simulink model "c166_ccp"  (Simulink 6.0)
settings: Solver=FixedStepDiscrete  StartTime=0.0  StopTime=16  FixedStep=0.01  RelTol=1e-3
PreLoadFcn:
  | c166_ccp_data
values from neighbouring files (symbols this model uses):
  STEP_PARAM = Simulink.Parameter    [c166_ccp_data.m]
undefined symbols (not defined in the file or in its folder): c166rt_ccp, Target_CCP
libraries: c166drivers x2
CloseFcn:
  | rtwprivate ssgencode ModelCloseRequest c166rt_ccp
settings Model: Creator=The MathWorks Inc.  LastModifiedBy=batserve  ExtModeAutoUpdateStatusClock=off  ProdHWDeviceType=Infineon C16x
settings DataIOCC: SignalLoggingName=logsOut
settings OptimizationCC: InlineParams=on  ZeroExternalMemoryAtStartup=off  ZeroInternalMemoryAtStartup=off  InitFltsAndDblsToZero=off  LifeSpan=1
settings DebuggingCC: CheckExecutionContextPreStartOutputMsg=on  CheckExecutionContextRuntimeOutputMsg=on  SignalResolutionControl=UseLocalSettings  SolverPrmCheckMsg=none
settings HardwareCC: ProdBitPerInt=16  ProdEndianess=LittleEndian  ProdWordSize=16  ProdHWDeviceType=Infineon C16x  TargetHWDeviceType=32-bit Generic
settings ModelReferenceCC: UpdateModelReferenceTargets=IfOutOfDate
settings RTWCC: SystemTargetFile=c166.tlc  TemplateMakefile=c166.tmf  ProcessScript=c166_make_rtw_hook
settings CodeAppCC: IgnoreCustomStorageClasses=off
settings STFCustomTargetCC: TargetFcnLib=ansi_tfl_tmw.mat  GenFloatMathFcnCalls=ANSI_C  GenerateSampleERTMain=on  CombineOutputUpdateFcns=on  ERTCustomFileBanners=on  SupportNonFinite=off  SystemTargetFile=c166.tlc
settings ERTTargetCC: TargetFcnLib=ansi_tfl_tmw.mat  GenFloatMathFcnCalls=ANSI_C  GenerateSampleERTMain=on  SupportNonFinite=off  SupportContinuousTime=on  SupportNonInlinedSFcns=on  GenerateASAP2=on  RootIOFormat=Individual Arguments  ERTCustomFileTemplate=example_file_process.tlc  InitialValueSource=Model
settings CustomProperty: DataType=RTWOptions_EnumType__toolbox_rtw_targets_c166_c166_c166_BuildActionC166  Value=None
settings EnumStrPairs: String=Run_with_simulator

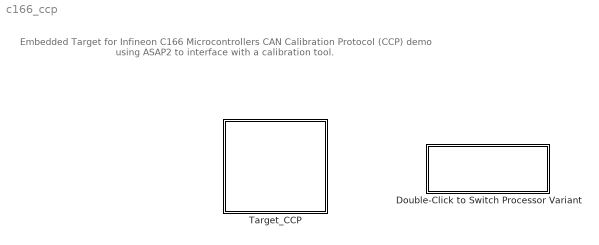
== system c166_ccp ==
  note: Embedded Target for Infineon C166 Microcontrollers
      | CAN Calibration Protocol (CCP) demo using
      | ASAP2 to interface with a calibration tool.
  Double-Click to Switch Processor Variant : Subsystem  PropExecContextAcrossSSBoundary=on
      settings: OpenFcn=c166switchconfig(gcs)
      mask Display: disp('Switch Target\nProcessor Variant');
  Target_CCP : Subsystem  InitFcn=|  PropExecContextAcrossSSBoundary=on
      | % START RTW CONFIGURATION CODE %
      | RTWConfigurationCB('rtw_target_initfcn',gcb);
      | % END RTW CONFIGURATION CODE %
      mask Display: image(imread('target_affordance_icon.jpg'),'bottom-right')

== system c166_ccp/Double-Click to Switch Processor Variant ==

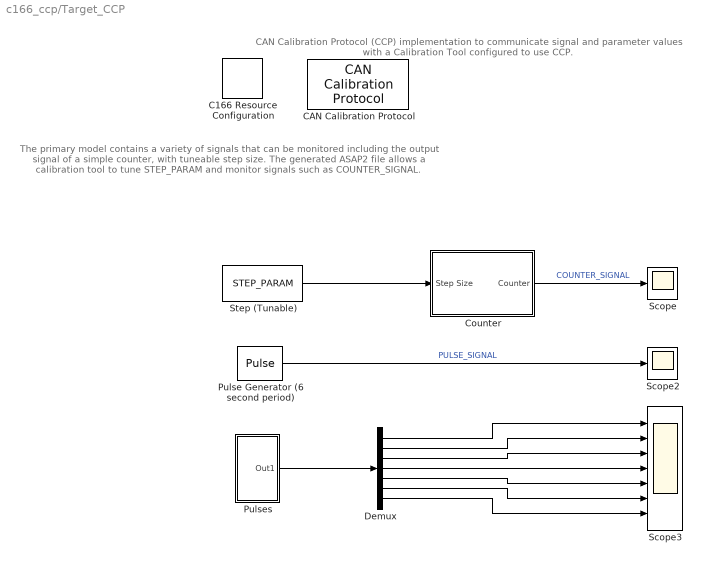
== system c166_ccp/Target_CCP ==
  note: The primary model contains a variety of signals that can be monitored
      | including the output signal of a simple counter, with tuneable
      | step size. The generated ASAP2 file allows a calibration tool to tune
      | STEP_PARAM and monitor signals such as COUNTER_SIGNAL.
  note: CAN Calibration Protocol (CCP) implementation
      | to communicate signal and parameter values
      |  with a Calibration Tool configured to use CCP.
  C166 Resource Configuration : c166drivers/C166 Resource Configuration  Tag=RTW CONFIGURATION BLOCK  Priority=-100000  oldParentName=c166rt_ccp/Target_CCP  oldBlockName=|  defaultConfigLibrary=c166drivers
      | c166rt_ccp/Target_CCP/C166
      | Resource
      | Configuration
  CAN Calibration Protocol : c166drivers/CAN Interface/CAN Calibration Protocol  CCP_STATION_ID=hex2dec('1')  module=A  ccp_cro_id=hex2dec('6FA')  ccp_cro_message_type=Extended (29-bit identifier)  ccp_return_id=hex2dec('6FB')  ccp_return_message_type=Extended (29-bit identifier)  TOTAL_NUM_ODTS=8  cro_sample_time=0.01
  Counter : Subsystem  PropExecContextAcrossSSBoundary=on
  Demux : Demux  Outputs=7
  Pulse Generator (6 second period) : DiscretePulseGenerator  Amplitude=uint16(60000)  Period=12  PulseWidth=4  SampleTime=0.5
  Pulses : Subsystem  PropExecContextAcrossSSBoundary=on
  Scope : Scope
      settings: YMin=-130  YMax=0
  Scope2 : Scope
      settings: YMin=-130  YMax=0  SaveName=ScopeData2
  Scope3 : Scope  NumInputPorts=7
      settings: YMin=-130~-5~-5~-5~-5~-5~-5  YMax=0~5~5~5~5~5~5  SaveName=ScopeData3
  Step (Tunable) : Constant  Value=STEP_PARAM
  wires:
  Step (Tunable)/1 -> Counter/1(Step Size)
  Counter/1(Counter) -> Scope/1  "COUNTER_SIGNAL"
  Pulse Generator (6 second period)/1 -> Scope2/1  "PULSE_SIGNAL"
  Pulses/1(Out1) -> Demux/1
  Demux/1 -> Scope3/1
  Demux/2 -> Scope3/2
  Demux/3 -> Scope3/3
  Demux/4 -> Scope3/4
  Demux/5 -> Scope3/5
  Demux/6 -> Scope3/6
  Demux/7 -> Scope3/7

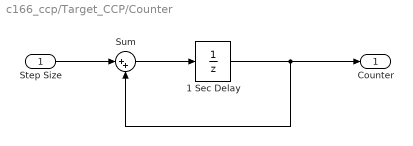
== system c166_ccp/Target_CCP/Counter ==
  Step Size : Inport  Port=1  LatchInput=off
  1 Sec Delay : UnitDelay
  Sum : Sum  Inputs=|++  SaturateOnIntegerOverflow=on  InputSameDT=on
  Counter : Outport
  wires:
  Sum/1 -> 1 Sec Delay/1
  1 Sec Delay/1 -> Sum/2, Counter/1
  Step Size/1 -> Sum/1

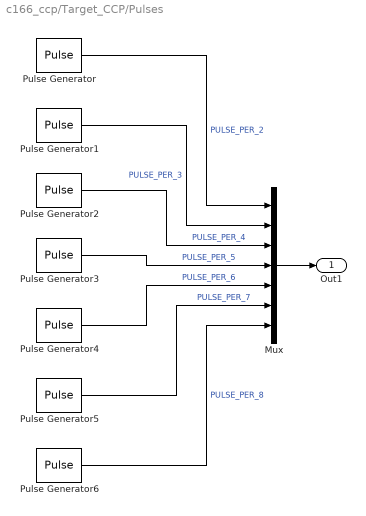
== system c166_ccp/Target_CCP/Pulses ==
  Mux : Mux  Inputs=7
  Pulse Generator : DiscretePulseGenerator  Amplitude=uint8(1)  SampleTime=0.1
  Pulse Generator1 : DiscretePulseGenerator  Amplitude=uint8(1)  Period=3  SampleTime=0.1
  Pulse Generator2 : DiscretePulseGenerator  Amplitude=uint8(1)  Period=4  SampleTime=0.1
  Pulse Generator3 : DiscretePulseGenerator  Amplitude=uint8(1)  Period=5  SampleTime=0.1
  Pulse Generator4 : DiscretePulseGenerator  Amplitude=uint8(1)  Period=6  SampleTime=0.1
  Pulse Generator5 : DiscretePulseGenerator  Amplitude=uint8(1)  Period=7  SampleTime=0.1
  Pulse Generator6 : DiscretePulseGenerator  Amplitude=uint8(1)  Period=8  SampleTime=0.1
  Out1 : Outport
  wires:
  Pulse Generator/1 -> Mux/1  "PULSE_PER_2"
  Pulse Generator1/1 -> Mux/2  "PULSE_PER_3"
  Pulse Generator2/1 -> Mux/3  "PULSE_PER_4"
  Pulse Generator3/1 -> Mux/4  "PULSE_PER_5"
  Pulse Generator4/1 -> Mux/5  "PULSE_PER_6"
  Pulse Generator5/1 -> Mux/6  "PULSE_PER_7"
  Pulse Generator6/1 -> Mux/7  "PULSE_PER_8"
  Mux/1 -> Out1/1
